simulink model "spikingneurons"  (R2021a)
settings: Solver=ode1  StartTime=0  StopTime=20  FixedStep=0.1  RelTol=1e-3
libraries: simulink x1
settings Model: Creator=runnily  LastModifiedBy=runnily

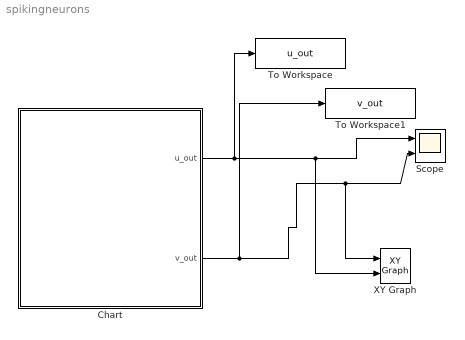
== system spikingneurons ==
  Chart : Stateflow chart  TreatAsAtomicUnit=on
  Scope : Scope  NumInputPorts=2
  To Workspace : ToWorkspace  VariableName=u_out  SaveFormat=Structure With Time  SampleTime=-1
  To Workspace1 : ToWorkspace  VariableName=v_out  SaveFormat=Structure With Time  SampleTime=-1
  XY Graph : simulink/Sinks/XY Graph  xmin=-100  xmax=100  ymin=-100  ymax=100  st=0.1
  wires:
  Chart/1(u_out) -> To Workspace/1, XY Graph/2, Scope/1
  Chart/2(v_out) -> To Workspace1/1, XY Graph/1, Scope/2

== stateflow chart spikingneurons/Chart ==
  settings: updateMethod=CONTINUOUS
  state spiking
    during:
    v_dot = 0.04 * v ^ 2 + 5 * v + 140 - u + 40;
    u_dot = 0.02 * (0.2 * v - u);
    v_out = v;
    u_out = u;
  (default) -> spiking : {v = 60.005; u = -0.215,  }
  spiking -> spiking : [v >= 30]{v = -65; u = u + 8}
  data: u_out output; v_out output; u local; v local
  data u settings: updateMethod=SF_CONTINUOUS_TIME_DATA
  data v settings: updateMethod=SF_CONTINUOUS_TIME_DATA
